simulink library "TSAA_AltRate_Error"  (R2016b)
settings: Solver=VariableStepAuto  StartTime=0.0  StopTime=10.0  RelTol=1e-3
undefined symbols (not defined in the file): randomSeed
settings Model: Creator=RA24876  LastModifiedBy=RA24876

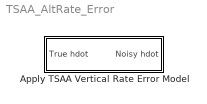
== system TSAA_AltRate_Error ==
  Apply TSAA Vertical Rate Error Model : Subsystem  mask{perfect=false, seed=randomSeed, dt_s=0}
      mask prompts: perfect "Use Perfect Altimetry?"; seed "randomSeed"; dt_s "Sample Time"

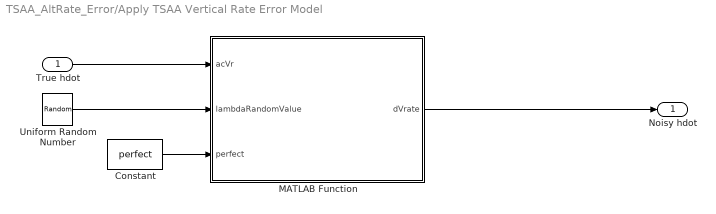
== system TSAA_AltRate_Error/Apply TSAA Vertical Rate Error Model ==
  True hdot : Inport
  Constant : Constant  Value=perfect
  MATLAB Function : MATLAB Function  TreatAsAtomicUnit=on
  Uniform Random Number : UniformRandomNumber  Minimum=0  Seed=seed  SampleTime=dt_s
  Noisy hdot : Outport
  wires:
  True hdot/1 -> MATLAB Function/1(acVr)
  Uniform Random Number/1 -> MATLAB Function/2(lambdaRandomValue)
  MATLAB Function/1(dVrate) -> Noisy hdot/1
  Constant/1 -> MATLAB Function/3(perfect)

== matlab function TSAA_AltRate_Error/Apply TSAA Vertical Rate Error Model/MATLAB Function ==
  data: acVr input; dVrate output; lambdaRandomValue input; perfect input
function dVrate  = degradeVrate(acVr, lambdaRandomValue, perfect)

dVrate = TSAA_Model_External_Functions.degradeVrate(acVr, lambdaRandomValue, perfect);
